simulink model "devStorageType12"  (R2018b)
settings: Solver=ode23  StartTime=0.0  StopTime=7000  MaxStep=300  RelTol=1e-3  EnableMultiTasking=on
undefined symbols (not defined in the file): path_carnot
libraries: carnot x8, simulink x5, Storage_Type_12 x1
settings Model: Creator=drhf  LastModifiedBy=drhf
settings DataIOCC: LimitDataPoints=on  SaveFormat=Array
settings OptimizationCC: ExpressionDepthLimit=2147483647  LifeSpan=inf
settings DebuggingCC: UnderspecifiedInitializationDetection=Classic  MergeDetectMultiDrivingBlocksExec=none  SolverPrmCheckMsg=warning  StateNameClashWarn=warning  SFUnexpectedBacktrackingDiag=warning  SFNoUnconditionalDefaultTransitionDiag=warning  SFExecutionAtInitializationDiag=none
settings HardwareCC: ProdBitPerPointer=32  ProdBitPerSizeT=32  ProdBitPerPtrDiffT=32  ProdLargestAtomicFloat=None  ProdIntDivRoundTo=Undefined  ProdEndianess=Unspecified  ProdWordSize=32  ProdHWDeviceType=32-bit Generic
settings ModelReferenceCC: PropagateSignalLabelsOutOfModel=off
settings SFSimCC: SimUseLocalCustomCode=off
settings RTWCC: RTWUseLocalCustomCode=off
settings CodeAppCC: StateflowObjectComments=on
settings GRTTargetCC: TargetLangStandard=C89/C90 (ANSI)  GeneratePreprocessorConditionals=Disable all  CombineOutputUpdateFcns=off  GRTInterface=on
settings ConfigComp: CovMetricSettings=dw  CovHtmlReporting=on  CovSaveCumulativeToWorkspaceVar=on  CovSaveSingleToWorkspaceVar=on  CovExternalEMLEnable=off

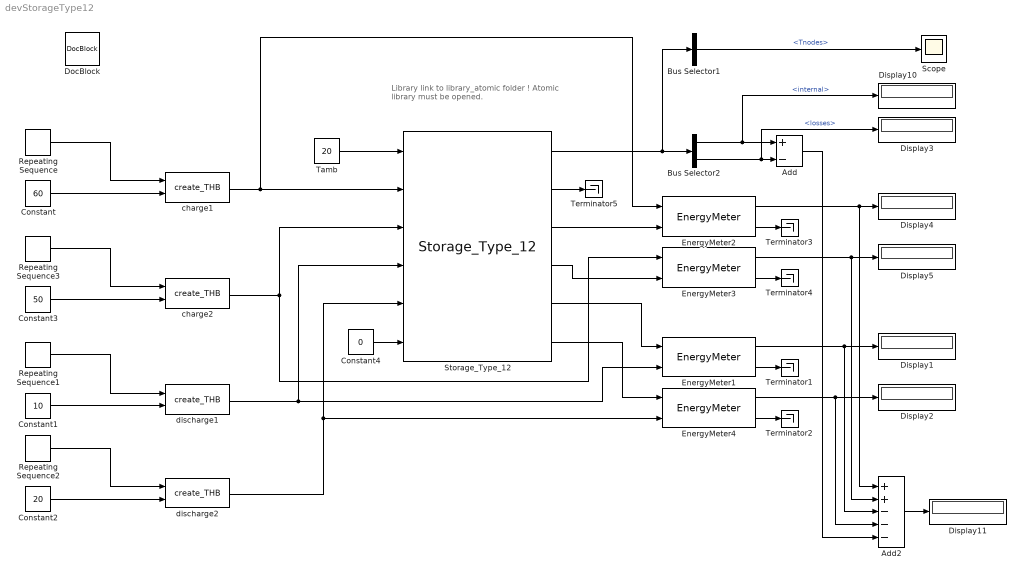
== system devStorageType12 ==
  note: Library link to library_atomic folder !
      | Atomic library must be opened.
  Add : Sum  Inputs=+-
  Add2 : Sum  Inputs=++---
  Bus Selector1 : BusSelector  OutputSignals=Tnodes
  Bus Selector2 : BusSelector  OutputSignals=energy.internal,energy.losses
  Constant : Constant  Value=60
  Constant1 : Constant  Value=10
  Constant2 : Constant  Value=20
  Constant3 : Constant  Value=50
  Constant4 : Constant  Value=0
  Display{1..5,10..11} (7 alike) : Display
  DocBlock : simulink/Model-Wide Utilities/DocBlock  DocumentType=Text
      content=|
      | This model is uses for the development of the block.
      | Open the corresponding atomic library to run the model (or add the folder
      | library_atomic to the Matlab path).
  EnergyMeter{1..4} (4 alike) : carnot/Control/EnergyMeter
      settings: SourceProductName=Carnot
  Repeating Sequence : simulink/Sources/Repeating Sequence  rep_seq_t=[0 1000 1010 7000]  rep_seq_y=[1 1 0 0]
  Repeating Sequence1 : simulink/Sources/Repeating Sequence  rep_seq_t=[0 1000 1010 2000 2010 7000]  rep_seq_y=[0 0 1 1 0 0]
  Repeating Sequence2 : simulink/Sources/Repeating Sequence  rep_seq_t=[0 5000 5010 6000 6010 7000]  rep_seq_y=[0 0 1.2 1.2 0 0]
  Repeating Sequence3 : simulink/Sources/Repeating Sequence  rep_seq_t=[0 3000 3010 4000 4010 7000]  rep_seq_y=[0 0 1 1 0 0]
  Scope : Scope
  Storage_Type_12 : Storage_Type_12/Storage_Type_12  t0=20  hgt=1.7684  stgtype=12  tini=[20 20 20 20 20 20 20 20 20 20]  mpts=[1 2 3 4 5 6 7 8 9 10]  PathName=fullfile(path_carnot('libsl'), 'Storage', 'Thermal', 'Storage_Type_12', 'parameter_set')  FileName='StorageType12_500_L.mat'  userPath=off  userParam=off  uwall=1  ubot=1  utop=1  axcond=1  volume=0.5  dia=0.6  standing=standing cylinder  nodes=10  mpoints=10  Tsensor=[0.2 0.4 0.6 0.8]  pipe1inlet=1  pipe1outlet=0  pipe1dia=0.05  pipe2inlet=1  pipe2outlet=0  pipe2dia=0.05  pipe3inlet=0  pipe3outlet=1  pipe3dia=0.05  pipe4inlet=0  pipe4outlet=1  pipe4dia=0.05  heater1start=0.6  heater1end=0.65
      settings: SourceProductName=Carnot
  Tamb : Constant  Value=20
  Terminator{1..5} (5 alike) : Terminator
  charge1 : carnot/Source/Simple/create_THB  p=1e5  fluid=Water  mix=0  mix2=0  mix3=0  dia=0  hgt=0  mID=No Pressure Drop
      settings: SourceProductName=Carnot
  charge2 : carnot/Source/Simple/create_THB  p=1e5  fluid=Water  mix=0  mix2=0  mix3=0  dia=0  hgt=0  mID=No Pressure Drop
      settings: SourceProductName=Carnot
  discharge1 : carnot/Source/Simple/create_THB  p=1e5  fluid=Water  mix=0  mix2=0  mix3=0  dia=0  hgt=0  mID=No Pressure Drop
      settings: SourceProductName=Carnot
  discharge2 : carnot/Source/Simple/create_THB  p=1e5  fluid=Water  mix=0  mix2=0  mix3=0  dia=0  hgt=0  mID=No Pressure Drop
      settings: SourceProductName=Carnot
  wires:
  Tamb/1 -> Storage_Type_12/1
  Storage_Type_12/1 -> Bus Selector1/1, Bus Selector2/1
  Storage_Type_12/2 -> Terminator5/1
  Add/1 -> Add2/5
  EnergyMeter3/1 -> Add2/2, Display5/1
  EnergyMeter3/2 -> Terminator4/1
  EnergyMeter2/1 -> Add2/1, Display4/1
  EnergyMeter2/2 -> Terminator3/1
  Add2/1 -> Display11/1
  Constant/1 -> charge1/2
  Repeating Sequence/1 -> charge1/1
  Repeating Sequence1/1 -> discharge1/1
  Constant1/1 -> discharge1/2
  Constant2/1 -> discharge2/2
  Repeating Sequence2/1 -> discharge2/1
  Constant3/1 -> charge2/2
  Repeating Sequence3/1 -> charge2/1
  charge1/1 -> Storage_Type_12/2, EnergyMeter2/1
  charge2/1 -> Storage_Type_12/3, EnergyMeter3/1
  discharge1/1 -> Storage_Type_12/4, EnergyMeter1/2
  discharge2/1 -> Storage_Type_12/5, EnergyMeter4/2
  Constant4/1 -> Storage_Type_12/6
  Storage_Type_12/3 -> EnergyMeter2/2
  EnergyMeter1/2 -> Terminator1/1
  EnergyMeter1/1 -> Add2/3, Display1/1
  EnergyMeter4/2 -> Terminator2/1
  EnergyMeter4/1 -> Add2/4, Display2/1
  Storage_Type_12/6 -> EnergyMeter4/1
  Bus Selector1/1 -> Scope/1  "<Tnodes>"
  Storage_Type_12/4 -> EnergyMeter3/2
  Storage_Type_12/5 -> EnergyMeter1/1
  Bus Selector2/1 -> Display10/1, Add/1  "<internal>"
  Bus Selector2/2 -> Display3/1, Add/2  "<losses>"
